simulink model "PubIfDecisionTOS_MDL"  (R2020b)
settings: configuration reference "DspaceConfig" (kept outside this file)
PostLoadFcn:
  | if any(exist('dsrtsu_mdlpostloadfcn', 'file') ~= 0), dsrtsu_mdlpostloadfcn('Execute', bdroot); end
InitFcn:
  | , if any(exist('dsmpb_private', 'file') ~= 0), dsmpb_private('dsmpb_mdlclblib', 'Init', bdroot); end,
undefined symbols (not defined in the file or in its folder): C_TOS_ACCEgoRAxletoFbumplength_m, C_TOS_ACCTargetFront_Flag, C_TOS_AEBJAPedObjDxThre_Val, C_TOS_AEBJAPedObjDyThre_Val, C_TOS_AEBJATargetSize_Val, C_TOS_AEBJAVehObjDxThre_Val, C_TOS_AEBJAVehObjDyThre_Val, C_TOS_AEBJuncPedTargetSize_Val, C_TOS_AEBLatObjDxThre_Val, C_TOS_AEBLatPedDyThre_Val, C_TOS_AEBLatTargetSize_Val, C_TOS_AEBLongTargetInEgoFront_Flag, C_TOS_axAbsGround_Parameter, C_TOS_CameraConfirmedFlag, C_TOS_CNsubjWidth, C_TOS_CurrentLaneCoreMinWidth_Val, C_TOS_CutInProb_Val_Zero, C_TOS_CutOutProb_Val_Zero, C_TOS_D2R_Val, C_TOS_DefaultValueObjectToCenterLine_dy, C_TOS_EgoCarWidth_Val, C_TOS_EgoDxRefPoint_m, C_TOS_EgoRAxletoFbumplength_m, C_TOS_HalfWidthVehicle_Con, C_TOS_HWA_CurrentLaneFlag, C_TOS_HWA_LeftLaneFlag, C_TOS_HWA_MovingDir_Vaild, C_TOS_HWA_MovState_Vaild, C_TOS_HWA_RightLaneFlag, C_TOS_LaneLineCourseErrorFront, C_TOS_LaneLineCourseErrorRear, C_TOS_MotorbikeDefaultWidth_m, C_TOS_NumberOfEffectiveTargets, C_TOS_Obj_Age_Val, C_TOS_Objdx_Constraint_Val, C_TOS_ObjectDefaultWidth_m, C_TOS_ObjInCurrentLane_Val, C_TOS_ObjInCurrentLaneValid, C_TOS_ObjInLeftLaneValid, C_TOS_ObjInRightLaneValid, C_TOS_ObjNotInCurrentLane_Val, C_TOS_ObjNotREElementType, C_TOS_ObjPredictDis_dy_ConstantVal_Zeros, C_TOS_ObjToCenterLine_ConstantVal_Zeros, C_TOS_OFMObjIDInvilad_Val, C_TOS_PIL_LatDisCons_Val_zero, C_TOS_PIL_ObjectCutInFlag_b, C_TOS_PIL_ObjectCutOutFlag_b, C_TOS_PIL_ObjLaneProb_al_Val, C_TOS_PP_ObjFusType_FC_Confirm_b, C_TOS_PP_ObjFusType_FC_FR_Confirm_b, C_TOS_PP_ObjFusType_FR_Confirm_b, C_TOS_RE_80BoolDefault_Val, C_TOS_RE_80Single181Default_Val, C_TOS_RE_80Single255Default_Val, C_TOS_RE_80Uint8Default_Val, C_TOS_RE_D2R, C_TOS_RE_D_180_Val, C_TOS_RE_InvalidObjectID_Val, C_TOS_RE_InvalidTargetChainDir_Val ... (+142)
libraries: simulink x1650, TOS_LIB x361, canfdmsglib x14
(part 6 of 69)

== system PubIfDecisionTOS_MDL/TOS_20201112/TOS_2012080320/PIL_1029/BoundaryCalculat/ObjectToCenterLine_dyc ==
  OFM_SignalVerification : Inport
  Left_CenterLine : Inport  Port=2
  Same_CenterLine : Inport  Port=3
  Right_CenterLine : Inport  Port=4
  Bus Creator1 : BusCreator  Inputs=4
  Bus Selector1 : BusSelector  OutputSignals=Left_CenterLine,OFM_SignalVerification
  Bus Selector2 : BusSelector  OutputSignals=Same_CenterLine,OFM_SignalVerification
  Bus Selector5 : BusSelector  OutputSignals=Right_CenterLine,OFM_SignalVerification
  LeftLane : Subsystem
  RightLane : Subsystem
  SameLane : Subsystem
  Terminator : Terminator
  Terminator1 : Terminator
  Terminator2 : Terminator
  PIL_LeftCenterLine_dyc_Filt : Outport
  PIL_SameCenterLine_dyc_Filt : Outport  Port=2
  PIL_RightCenterLine_dyc_Filt : Outport  Port=3
  wires:
  Left_CenterLine/1 -> Bus Creator1/2  "Left_CenterLine"
  Same_CenterLine/1 -> Bus Creator1/3  "Same_CenterLine"
  Bus Creator1/1 -> Bus Selector1/1, Bus Selector2/1, Bus Selector5/1
  Bus Selector2/1 -> SameLane/1(Same_CenterLine)  "<Same_CenterLine>"
  Bus Selector2/2 -> SameLane/2(OFM_SignalVerification)  "<OFM_SignalVerification>"
  SameLane/1(PIL_SameCenterLine_dyc) -> Terminator1/1  "PIL_SameCenterLine_dyc"
  LeftLane/1(PIL_LeftCenterLine_dyc) -> Terminator/1  "PIL_LeftCenterLine_dyc"
  Bus Selector1/1 -> LeftLane/1(Left_CenterLine)  "<Left_CenterLine>"
  Bus Selector1/2 -> LeftLane/2(OFM_SignalVerification)  "<OFM_SignalVerification>"
  RightLane/1(PIL_RightCenterLine_dyc) -> Terminator2/1  "PIL_RightCenterLine_dyc"
  Right_CenterLine/1 -> Bus Creator1/4  "Right_CenterLine"
  OFM_SignalVerification/1 -> Bus Creator1/1  "OFM_SignalVerification"
  Bus Selector5/2 -> RightLane/2(OFM_SignalVerification)  "<OFM_SignalVerification>"
  Bus Selector5/1 -> RightLane/1(CenterOfRightLane)  "<Right_CenterLine>"
  LeftLane/2(PIL_LeftCenterLine_dyc_Filt) -> PIL_LeftCenterLine_dyc_Filt/1
  SameLane/2(PIL_SameCenterLine_dyc_Filt) -> PIL_SameCenterLine_dyc_Filt/1
  RightLane/2(PIL_RightCenterLine_dyc_Filt) -> PIL_RightCenterLine_dyc_Filt/1

== system PubIfDecisionTOS_MDL/TOS_20201112/TOS_2012080320/PIL_1029/ObjCutInOut_Prob/ObjectCutIn ==
  TOS_OFMObjValid_Flag : Inport
  Object_Width : Inport  Port=2  OutDataTypeStr=single
  Object_DX : Inport  Port=3  OutDataTypeStr=single
  Object_DY : Inport  Port=4  OutDataTypeStr=single
  Object_Age : Inport  Port=5  OutDataTypeStr=uint16
  Object_Type : Inport  Port=6
  Object_MovingState : Inport  Port=7
  PP_ObjectToCenterLine_dy : Inport  Port=8  OutDataTypeStr=single
  PP_ObjectToCenterLine_vyc : Inport  Port=9  OutDataTypeStr=single
  PP_CurrentLaneWidth : Inport  Port=10
  PIL_ObjectToCenterLine_dy_Filt : Inport  Port=11  OutDataTypeStr=single
  Bus Creator : BusCreator  Inputs=11
  Bus Creator1 : BusCreator  Inputs=5
  Bus Selector : BusSelector  OutputSignals=TOS_OFMObjValid_Flag,Object_Width,Object_DX,Object_DY,Object_Age,Object_Type,PP_ObjectToCenterLine_dy,PP_ObjectToCenterLine_vyc,PIL_ObjectToCenterLine_dy_Filt,PP_CurrentLaneWidth
  Bus Selector4 : BusSelector  OutputSignals=Object_DX,TOS_OFMObjValid_Flag,Object_MovingState
  CutInProb_Calculate : Subsystem
  CutInProb_Pluse : Subsystem
  Terminator : Terminator
  Unit Delay : UnitDelay  InitialCondition=zeros(80,1)  SampleTime=-1  HasFrameUpgradeWarning=on
  TOS_PIL_ObjectCutInPro_Filt : Outport
  TOS_PIL_ObjectCutIn_Flag : Outport  Port=2
  wires:
  Bus Creator1/1 -> Terminator/1  "TOS_PIL_Cutin_ObserVale"
  Bus Selector4/3 -> CutInProb_Pluse/5(Object_MovingState)  "<Object_MovingState>"
  Object_MovingState/1 -> Bus Creator/7  "Object_MovingState"
  CutInProb_Pluse/1(PIL_CutInProb_Pluse) -> TOS_PIL_ObjectCutInPro_Filt/1, Unit Delay/1  "TOS_PIL_ObjectCutInPro_Filt"
  CutInProb_Pluse/2(PIL_ObjectCutInFlag) -> TOS_PIL_ObjectCutIn_Flag/1  "TOS_PIL_ObjectCutIn_Flag"
  Object_Width/1 -> Bus Creator/2  "Object_Width"
  Object_DX/1 -> Bus Creator/3  "Object_DX"
  Object_DY/1 -> Bus Creator/4  "Object_DY"
  Object_Age/1 -> Bus Creator/5  "Object_Age"
  PP_ObjectToCenterLine_dy/1 -> Bus Creator/8  "PP_ObjectToCenterLine_dy"
  PP_ObjectToCenterLine_vyc/1 -> Bus Creator/9  "PP_ObjectToCenterLine_vyc"
  PIL_ObjectToCenterLine_dy_Filt/1 -> Bus Creator/11  "PIL_ObjectToCenterLine_dy_Filt"
  Bus Creator/1 -> Bus Selector/1, [ObjCutInSig]
  Unit Delay/1 -> CutInProb_Pluse/1(CutInProb_Pluse_K1)
  Object_Type/1 -> Bus Creator/6  "Object_Type"
  PP_CurrentLaneWidth/1 -> Bus Creator/10  "PP_CurrentLaneWidth"
  Bus Selector4/1 -> CutInProb_Pluse/3(Object_Dx)  "<Object_DX>"
  [ObjCutInSig] -> Bus Selector4/1
  CutInProb_Calculate/5(CutInProb_Calculate) -> Bus Creator1/5, CutInProb_Pluse/2(CutInProb_ScopeConstraint)  "TOS_PIL_CutInProb_Calculate"
  Bus Selector/2 -> CutInProb_Calculate/2(Object_Width)  "<Object_Width>"
  Bus Selector/3 -> CutInProb_Calculate/3(Object_DX)  "<Object_DX>"
  Bus Selector/4 -> CutInProb_Calculate/4(Object_DY)  "<Object_DY>"
  Bus Selector/5 -> CutInProb_Calculate/5(Object_Age)  "<Object_Age>"
  Bus Selector/6 -> CutInProb_Calculate/6(Object_Type)  "<Object_Type>"
  Bus Selector/7 -> CutInProb_Calculate/7(PP_ObjectToCenterLine_dy)  "<PP_ObjectToCenterLine_dy>"
  Bus Selector/8 -> CutInProb_Calculate/8(PP_ObjectToCenterLine_vyc)  "<PP_ObjectToCenterLine_vyc>"
  Bus Selector/9 -> CutInProb_Calculate/9(PIL_ObjectToCenterLine_dy_Filt)  "<PIL_ObjectToCenterLine_dy_Filt>"
  Bus Selector/10 -> CutInProb_Calculate/10(PP_CurrentLaneWidth)  "<PP_CurrentLaneWidth>"
  CutInProb_Calculate/1(PIL_CutInPredictTime_ObserVale) -> Bus Creator1/1  "TOS_PIL_CutInPredictTime_ObserVale"
  CutInProb_Calculate/2(PIL_CutInPredictTime_dxConstraint_ObserVale) -> Bus Creator1/2  "TOS_PIL_CutInPredictTime_dxConstraint_ObserVale"
  CutInProb_Calculate/3(PIL_CutInPredictDis_dy_ObjWidthConstraint_ObserVale) -> Bus Creator1/3  "TOS_PIL_CutInPredictDis_dy_ObjWidthConstraint_ObserVale"
  CutInProb_Calculate/4(PIL_ObjectCutinMindFlg_ObserVale) -> Bus Creator1/4  "TOS_PIL_CutinMindFlg_ObserVale"
  TOS_OFMObjValid_Flag/1 -> Bus Creator/1  "TOS_OFMObjValid_Flag"
  Bus Selector/1 -> CutInProb_Calculate/1(TOS_OFMObjValid_Flag)  "<TOS_OFMObjValid_Flag>"
  Bus Selector4/2 -> CutInProb_Pluse/4(TOS_OFMObjValid_Flag)  "<TOS_OFMObjValid_Flag>"

== system PubIfDecisionTOS_MDL/TOS_20201112/TOS_2012080320/PIL_1029/ObjCutInOut_Prob/ObjectCutOut ==
  TOS_OFMObjValid_Flag : Inport
  Object_Width : Inport  Port=2
  Object_DX : Inport  Port=3
  Object_DY : Inport  Port=4
  Object_Age : Inport  Port=5
  Object_Type : Inport  Port=6
  Object_MovingState : Inport  Port=7
  Object_VY : Inport  Port=8
  Object_Std_DY : Inport  Port=9
  PP_ObjectToCenterLine_dy : Inport  Port=10
  PP_ObjectToCenterLine_vyc : Inport  Port=11
  PIL_ObjectToCenterLine_dy_Filt : Inport  Port=12
  Bus Creator : BusCreator  Inputs=11
  Bus Creator1 : BusCreator  Inputs=7
  Bus Selector : BusSelector  OutputSignals=TOS_OFMObjValid_Flag,Object_Width,Object_DX,Object_DY,Object_Age,Object_Type,PP_ObjectToCenterLine_dy,PP_ObjectToCenterLine_vyc,PIL_ObjectToCenterLine_dy_Filt,Object_VY
  Bus Selector4 : BusSelector  OutputSignals=TOS_OFMObjValid_Flag,Object_MovingState
  CutOutProb_Calculate : Subsystem
  CutOutProb_Pluse : Subsystem
  Subsystem : Subsystem
  Terminator : Terminator
  Terminator1 : Terminator
  Unit Delay : UnitDelay  InitialCondition=zeros(80,1)  SampleTime=-1  HasFrameUpgradeWarning=on
      settings: AttributesFormatString=initVal = zeros(80,1)
  TOS_PIL_ObjectCutOutPro_Filt : Outport
  TOS_PIL_ObjectCutOut_Flag : Outport  Port=2
  wires:
  Subsystem/1(Out1) -> CutOutProb_Calculate/10(Object_VY)  "OBJ_VY"
  Bus Selector/10 -> Subsystem/1(In1)  "<Object_VY>"
  Object_VY/1 -> Bus Creator/11  "Object_VY"
  Bus Selector4/2 -> CutOutProb_Pluse/4(Object_MovingState)  "<Object_MovingState>"
  Object_MovingState/1 -> Bus Creator/10  "Object_MovingState"
  Unit Delay/1 -> CutOutProb_Pluse/1(CutOutProb_Pluse_K1)
  CutOutProb_Pluse/2(PIL_ObjectCutOutFlag) -> TOS_PIL_ObjectCutOut_Flag/1  "TOS_PIL_ObjectCutOut_Flag"
  CutOutProb_Pluse/1(PIL_CutOutProb_Pluse) -> Unit Delay/1, TOS_PIL_ObjectCutOutPro_Filt/1  "TOS_PIL_ObjectCutOutPro_Filt"
  CutOutProb_Calculate/1(PIL_CutOutPredictTime_ObserVale) -> Bus Creator1/1  "TOS_PIL_CutOutPredictTime_ObserVale"
  CutOutProb_Calculate/2(PIL_CutOutPredictTime_dxConstraint_ObserVale) -> Bus Creator1/2  "TOS_PIL_CutOutPredictTime_dxConstraint_ObserVale"
  CutOutProb_Calculate/3(PIL_CutOutPredictDis_dy_ObjWidthConstraint_ObserVale) -> Bus Creator1/3  "TOS_CutOutPredictDis_dy_ObjWidthConstraint_ObserVale"
  CutOutProb_Calculate/4(PIL_ObjectCutOutMindFlg_ObserVale) -> Bus Creator1/4  "TOS_PIL_ObjectCutOutMindFlg_ObserVale"
  CutOutProb_Calculate/8(PIL_CutOutProb_ScopeConstraint) -> CutOutProb_Pluse/2(CutOutProb_ScopeConstraint)
  Bus Creator/1 -> Bus Selector/1, [ObjectCutOut]
  TOS_OFMObjValid_Flag/1 -> Bus Creator/1  "TOS_OFMObjValid_Flag"
  Object_Width/1 -> Bus Creator/2  "Object_Width"
  Object_DX/1 -> Bus Creator/3  "Object_DX"
  Object_DY/1 -> Bus Creator/4  "Object_DY"
  Object_Age/1 -> Bus Creator/5  "Object_Age"
  Object_Type/1 -> Bus Creator/6  "Object_Type"
  PP_ObjectToCenterLine_dy/1 -> Bus Creator/7  "PP_ObjectToCenterLine_dy"
  PP_ObjectToCenterLine_vyc/1 -> Bus Creator/8  "PP_ObjectToCenterLine_vyc"
  PIL_ObjectToCenterLine_dy_Filt/1 -> Bus Creator/9  "PIL_ObjectToCenterLine_dy_Filt"
  Bus Selector/1 -> CutOutProb_Calculate/1(TOS_OFMObjValid_Flag)  "<TOS_OFMObjValid_Flag>"
  Bus Selector/2 -> CutOutProb_Calculate/2(Object_Width)  "<Object_Width>"
  Bus Selector/3 -> CutOutProb_Calculate/3(Object_DX)  "<Object_DX>"
  Bus Selector/4 -> CutOutProb_Calculate/4(Object_DY)  "<Object_DY>"
  Bus Selector/5 -> CutOutProb_Calculate/5(Object_Age)  "<Object_Age>"
  Bus Selector/6 -> CutOutProb_Calculate/6(Object_Type)  "<Object_Type>"
  Bus Selector/7 -> CutOutProb_Calculate/7(PP_ObjectToCenterLine_dy)  "<PP_ObjectToCenterLine_dy>"
  Bus Selector/8 -> CutOutProb_Calculate/8(PP_ObjectToCenterLine_vyc)  "<PP_ObjectToCenterLine_vyc>"
  Bus Selector/9 -> CutOutProb_Calculate/9(PIL_ObjectToCenterLine_dy_Filt)  "<PIL_ObjectToCenterLine_dy_Filt>"
  [ObjectCutOut] -> Bus Selector4/1
  Bus Selector4/1 -> CutOutProb_Pluse/3(TOS_OFMObjValid_Flag)  "<TOS_OFMObjValid_Flag>"
  Object_Std_DY/1 -> Terminator/1
  CutOutProb_Calculate/5(PIL_ObjectCutoutMindFlg1_ObserVale) -> Bus Creator1/5  "TOS_PIL_ObjectCutoutMindFlg1_ObserVale"
  CutOutProb_Calculate/6(PIL_ObjectCutoutMindFlg2_ObserVale) -> Bus Creator1/6  "TOS_PIL_ObjectCutoutMindFlg2_ObserVale"
  CutOutProb_Calculate/7(PIL_ObjectCutoutMindFlg3_ObserVale) -> Bus Creator1/7  "TOS_PIL_ObjectCutoutMindFlg3_ObserVale"
  Bus Creator1/1 -> Terminator1/1  "TOS_PIL_CutOut_ObserVale"

== system PubIfDecisionTOS_MDL/TOS_20201112/TOS_2012080320/PIL_1029/OverlapRatio_Calculate/OverlapCalculation_Default ==
  Action Port : ActionPort  ActionPortLabel=if(u1 ~= 0)
  Constant2 : Constant  Value=0  OutDataTypeStr=single
  PIL_overlapRatio : Outport  OutDataTypeStr=single
  wires:
  Constant2/1 -> PIL_overlapRatio/1

== system PubIfDecisionTOS_MDL/TOS_20201112/TOS_2012080320/PIL_1029/OverlapRatio_Calculate/PIL_OverlapCalculation ==
  ObjectWidth : Inport
  ObjectTypeCameraConfirmed : Inport  Port=2
  object_MovingState : Inport  Port=3
  Object_Type : Inport  Port=4
  dyEgo2Center : Inport  Port=5
  dyObject2Center : Inport  Port=6
  Action Port : ActionPort  ActionPortLabel=else
  OverlapRatioCalcFlow : Stateflow chart  TreatAsAtomicUnit=on
  TargetWidthCalc : Subsystem
  dyCriticalEgoObjCalc : Subsystem
  overlapRatio : Outport
  wires:
  dyObject2Center/1 -> OverlapRatioCalcFlow/3(dyObject2Center)
  dyEgo2Center/1 -> OverlapRatioCalcFlow/2(dyEgo2Center)
  OverlapRatioCalcFlow/1(overlapRatio) -> overlapRatio/1
  dyCriticalEgoObjCalc/1(dyCriticalEgoObj) -> OverlapRatioCalcFlow/1(dyCriticalEgoObj)  "dyCriticalEgoObj"
  TargetWidthCalc/1(objWidth) -> dyCriticalEgoObjCalc/1(objWidth)  "objWidth"
  object_MovingState/1 -> TargetWidthCalc/3(object_MovingState)
  ObjectTypeCameraConfirmed/1 -> TargetWidthCalc/2(ObjectTypeCameraConfirmed)
  ObjectWidth/1 -> TargetWidthCalc/1(ObjectWidth)
  Object_Type/1 -> TargetWidthCalc/4(Object_Type)

== system PubIfDecisionTOS_MDL/TOS_20201112/TOS_2012080320/PIL_1029/PIL_ObjectToCenterLine_dy_Filt/PIL_ObjectToCenterLine_dy ==
  ObjectID_Filt_K1 : Inport
  ObjectToCenterLine_dy_Filt_K1 : Inport  Port=2  OutDataTypeStr=single
  ObjectToCenterLine_dy : Inport  Port=3  OutDataTypeStr=single  Partition=on  PartitionDimension=1  PartitionWidth=1  PartitionOffset=0
  TOS_OFMObjValid_Flag : Inport  Port=4  OutDataTypeStr=uint8  Partition=on  PartitionDimension=1  PartitionWidth=1  PartitionOffset=0
  Object_ID : Inport  Port=5  OutDataTypeStr=uint8  Partition=on  PartitionDimension=1  PartitionWidth=1  PartitionOffset=0
  Object_Age : Inport  Port=6  Partition=on  PartitionDimension=1  PartitionWidth=1  PartitionOffset=0
  Compare To Constant : simulink/Logic and Bit Operations/Compare To Constant  relop===  const=C_TOS_OFMObjIDInvilad_Val  OutDataTypeStr=boolean
      settings: AttributesFormatString=C_TOS_OFMObjIDInvilad_Val = 0
  For Each : ForEach  DisableCoverage=on
  If : If  IfExpression=u1 ~= 0
  Merge : Merge
  Merge1 : Merge
  PP_SignalProcessingDefault : Subsystem  TreatAsAtomicUnit=on
  Subsystem : Subsystem
  Obj_ID : Outport  ConcatenationDimension=1
  ObjectToCenterLine_dy_Filt : Outport  Port=2  OutDataTypeStr=single  ConcatenationDimension=1
  wires:
  [TOS_OFMObjValid_Flag] -> Subsystem/6(TOS_OFMObjValid_Flag)
  TOS_OFMObjValid_Flag/1 -> Compare To Constant/1, [TOS_OFMObjValid_Flag]
  Object_Age/1 -> Subsystem/5(Object_Age)
  Merge/1 -> Obj_ID/1
  Merge1/1 -> ObjectToCenterLine_dy_Filt/1
  PP_SignalProcessingDefault/2(ObjectToCenterLine_dy_Filt) -> Merge1/1
  PP_SignalProcessingDefault/1(Obj_ID) -> Merge/1
  Subsystem/2(ObjectToCenterLine_dy_Filt) -> Merge1/2
  Subsystem/1(Obj_ID) -> Merge/2
  ObjectToCenterLine_dy/1 -> Subsystem/3(ObjectToCenterLine_dy)
  ObjectToCenterLine_dy_Filt_K1/1 -> Subsystem/2(ObjectToCenterLine_dy_Filt_K1)
  ObjectID_Filt_K1/1 -> Subsystem/1(ObjectID_Filt_K1)
  Compare To Constant/1 -> If/1
  Object_ID/1 -> Subsystem/4(Object_ID)
  If/1 -> PP_SignalProcessingDefault/Action
  If/2 -> Subsystem/Action

== system PubIfDecisionTOS_MDL/TOS_20201112/TOS_2012080320/PIL_1029/ProbCalculat/ProbCalculat ==
  OFM_SignalVerification : Inport
  CurrentLane_Boundary : Inport  Port=2
  PIL_ObjectToCenterLine_dyc : Inport  Port=3
  LM_SignalVerification : Inport  Port=4
  Bus Selector1 : BusSelector  OutputSignals=PIL_SameCenterLine_dyc,PIL_LeftCenterLine_dyc,PIL_RightCenterLine_dyc
  Bus Selector2 : BusSelector  OutputSignals=SameLane_CoreArea_Boundary,SameLane_EdgeLeft_Boundary,SameLane_EdgeRight_Boundary,LeftLane_CoreArea_Boundary,LeftLane_EdgeLeft_Boundary,LeftLane_EdgeRight_Boundary,RightLane_CoreArea_Boundary,RightLane_EdgeLeft_Boundary,RightLane_EdgeRight_Boundary
  Bus Selector3 : BusSelector  OutputSignals=TOS_OFMObjValid_Flag,Object_Width,Object_Type
  ObjectProbCalculation : Subsystem
  Subsystem : Subsystem
  PIL_EgoLaneProb : Outport  InitialOutput=0
  PIL_LeftLaneProb : Outport  Port=2
  PIL_RightLaneProb : Outport  Port=3
  "PIL_ObjLaneProb_all " : Outport  Port=4  InitialOutput=0
  PIL_EgoVehicleProFilt : Outport  Port=5
  wires:
  Bus Selector2/9 -> ObjectProbCalculation/15(RightLane_EdgeRight_Boundary)  "<RightLane_EdgeRight_Boundary>"
  Bus Selector2/8 -> ObjectProbCalculation/14(RightLane_EdgeLeft_Boundary)  "<RightLane_EdgeLeft_Boundary>"
  Bus Selector2/7 -> ObjectProbCalculation/13(RightLane_CoreArea_Boundary)  "<RightLane_CoreArea_Boundary>"
  Bus Selector2/6 -> ObjectProbCalculation/12(LeftLane_EdgeRight_Boundary)  "<LeftLane_EdgeRight_Boundary>"
  Bus Selector2/5 -> ObjectProbCalculation/11(LeftLane_EdgeLeft_Boundary)  "<LeftLane_EdgeLeft_Boundary>"
  Bus Selector2/4 -> ObjectProbCalculation/10(LeftLane_CoreArea_Boundary)  "<LeftLane_CoreArea_Boundary>"
  Bus Selector1/3 -> ObjectProbCalculation/6(PIL_RightCenterLine_dyc)  "<PIL_RightCenterLine_dyc>"
  Bus Selector1/2 -> ObjectProbCalculation/5(PIL_LeftCenterLine_dyc)  "<PIL_LeftCenterLine_dyc>"
  Bus Selector1/1 -> ObjectProbCalculation/4(PIL_SameCenterLine_dyc)  "<PIL_SameCenterLine_dyc>"
  PIL_ObjectToCenterLine_dyc/1 -> Bus Selector1/1
  Bus Selector2/2 -> ObjectProbCalculation/8(SameLane_EdgeLeft_Boundary)  "<SameLane_EdgeLeft_Boundary>"
  Bus Selector2/3 -> ObjectProbCalculation/9(SameLane_EdgeRight_Boundary)  "<SameLane_EdgeRight_Boundary>"
  Bus Selector2/1 -> ObjectProbCalculation/7(SameLane_CoreArea_Boundary)  "<SameLane_CoreArea_Boundary>"
  Bus Selector3/3 -> ObjectProbCalculation/3(Object_Type)  "<Object_Type>"
  Bus Selector3/2 -> ObjectProbCalculation/2(Object_Width)  "<Object_Width>"
  Bus Selector3/1 -> ObjectProbCalculation/1(TOS_OFMObjValid_Flag)  "<TOS_OFMObjValid_Flag>"
  CurrentLane_Boundary/1 -> Bus Selector2/1
  OFM_SignalVerification/1 -> Bus Selector3/1
  LM_SignalVerification/1 -> Subsystem/1(LM_SignalVerification)
  Subsystem/1(PIL_EgoVehicleProFilt) -> PIL_EgoVehicleProFilt/1
  ObjectProbCalculation/1("PIL_ObjLaneProb_all ") -> "PIL_ObjLaneProb_all "/1  "PIL_ObjLaneProb_all"
  ObjectProbCalculation/2(PIL_EgoLaneProb) -> PIL_EgoLaneProb/1  "PIL_EgoLaneProb"
  ObjectProbCalculation/3(PIL_LeftLaneProb) -> PIL_LeftLaneProb/1  "PIL_LeftLaneProb"
  ObjectProbCalculation/4(PIL_RightLaneProb) -> PIL_RightLaneProb/1  "PIL_RightLaneProb"

== system PubIfDecisionTOS_MDL/TOS_20201112/TOS_2012080320/PIL_1029/ProbCalculat/ProbFilt ==
  OFM_InPutSig : Inport
  PIL_ObjinEgoLaneProb : Inport  Port=2
  PIL_ObjinLeftLaneProb : Inport  Port=3
  PIL_ObjinRightLaneProb : Inport  Port=4
  ObjinEgoLaneProb : Subsystem
  ObjinLeftLaneProb : Subsystem
  ObjinRightLaneProb : Subsystem
  Signal Copy : SignalConversion  OverrideOpt=off
  Signal Copy1 : SignalConversion  OverrideOpt=off
  Signal Copy2 : SignalConversion  OverrideOpt=off
  Terminator : Terminator
  PIL_ObjinEgoLaneProb_Filt : Outport
  PIL_ObjinLeftLaneProb_Filt : Outport  Port=2
  PIL_ObjinRightLaneProb_Filt : Outport  Port=3
  wires:
  ObjinRightLaneProb/1(PIL_ObjinRightLaneProb_Filt) -> Signal Copy/1
  ObjinLeftLaneProb/1(PIL_ObjinLeftLaneProb_Filt) -> Signal Copy1/1
  ObjinEgoLaneProb/1(PIL_ObjinEgoLaneProb_Filt) -> Signal Copy2/1
  Signal Copy/1 -> PIL_ObjinRightLaneProb_Filt/1  "TOS_PIL_RightLaneProb_Filt"
  Signal Copy1/1 -> PIL_ObjinLeftLaneProb_Filt/1  "TOS_PIL_LeftLaneProb_Filt"
  Signal Copy2/1 -> PIL_ObjinEgoLaneProb_Filt/1  "TOS_PIL_SameLanePro_Filt"
  PIL_ObjinEgoLaneProb/1 -> ObjinEgoLaneProb/1(PIL_ObjinEgoLaneProb)
  PIL_ObjinLeftLaneProb/1 -> ObjinLeftLaneProb/1(PIL_ObjinLeftLaneProb)
  PIL_ObjinRightLaneProb/1 -> ObjinRightLaneProb/1(PIL_ObjinRightLaneProb)
  OFM_InPutSig/1 -> Terminator/1

== system PubIfDecisionTOS_MDL/TOS_20201112/TOS_2012080320/PP1128/AAT-AdditionalAttributes/PP_CenterLine_Calculat ==
  OFM_SignalVerification : Inport
  LM_SignalVerification : Inport  Port=2
  EgoLane_CenterLine : Subsystem
  LaneWidth : Subsystem
  LaneWidth_80 : Subsystem  Commented=on
  LeftLane_CenterLine : Subsystem
  RightLane_CenterLine : Subsystem
  Terminator : Terminator  Commented=on
  PP_EgoLane_CenterLine : Outport
  PP_LeftLane_CenterLine : Outport  Port=2
  PP_RightLane_CenterLine : Outport  Port=3
  PP_LaneWidth : Outport  Port=4
  wires:
  LM_SignalVerification/1 -> EgoLane_CenterLine/1(EgoLane), RightLane_CenterLine/1(LeftLane), LeftLane_CenterLine/1(LeftLane), LaneWidth/1(LM_SignalVerification), LaneWidth_80/2(LM_SignalVerification)
  EgoLane_CenterLine/1(PP_EgoLane_CenterLine) -> PP_EgoLane_CenterLine/1
  LeftLane_CenterLine/1(PP_LeftLane_CenterLine) -> PP_LeftLane_CenterLine/1
  RightLane_CenterLine/1(PP_RightLane_CenterLine) -> PP_RightLane_CenterLine/1
  LaneWidth/1(PP_LaneWidth) -> PP_LaneWidth/1
  OFM_SignalVerification/1 -> LaneWidth_80/1(OFM_SignalVerification)
  LaneWidth_80/1(PP_LaneWidth) -> Terminator/1

== system PubIfDecisionTOS_MDL/TOS_20201112/TOS_2012080320/PP1128/AAT-AdditionalAttributes/PP_ObjFirstDxDyDetermineSignalProcessing ==
  Object_DX : Inport
  Object_DY : Inport  Port=2
  Object_ID : Inport  Port=3
  TOS_OFMObjValid_Flag : Inport  Port=4
  PP_ObjFirstDxDyDetermine : Subsystem
  Unit Delay : UnitDelay  InitialCondition=zeros(80,1)  SampleTime=-1  HasFrameUpgradeWarning=on
      settings: AttributesFormatString=initVal = zeros(80,1)
  Unit Delay1 : UnitDelay  InitialCondition=zeros(80,1)  SampleTime=-1  HasFrameUpgradeWarning=on
      settings: AttributesFormatString=initVal = zeros(80,1)
  Unit Delay2 : UnitDelay  InitialCondition=zeros(80,1)  SampleTime=-1  HasFrameUpgradeWarning=on
      settings: AttributesFormatString=initVal = zeros(80,1)
  PP_ObjFirstDetect_Dx : Outport
  PP_ObjFirstDetect_Dy : Outport  Port=2
  wires:
  Unit Delay2/1 -> PP_ObjFirstDxDyDetermine/1(Object_ID_Last)
  PP_ObjFirstDxDyDetermine/3(PP_ObjFirstDetect_Dy) -> Unit Delay/1, PP_ObjFirstDetect_Dy/1
  PP_ObjFirstDxDyDetermine/1(Object_ID_temp) -> Unit Delay2/1
  Unit Delay/1 -> PP_ObjFirstDxDyDetermine/3(Object_Dy_Last)
  PP_ObjFirstDxDyDetermine/2(PP_ObjFirstDetect_Dx) -> Unit Delay1/1, PP_ObjFirstDetect_Dx/1
  Unit Delay1/1 -> PP_ObjFirstDxDyDetermine/2(Object_Dx_Last)
  Object_DX/1 -> PP_ObjFirstDxDyDetermine/4(Object_Dx)
  Object_DY/1 -> PP_ObjFirstDxDyDetermine/5(Object_Dy)
  Object_ID/1 -> PP_ObjFirstDxDyDetermine/6(Object_ID)
  TOS_OFMObjValid_Flag/1 -> PP_ObjFirstDxDyDetermine/7(TOS_OFMObjValid_Flag)

== system PubIfDecisionTOS_MDL/TOS_20201112/TOS_2012080320/PP1128/AAT-AdditionalAttributes/PP_ObjectToCenterLine_dy ==
  "OFM_SignalVerification " : Inport
  LM_SignalVerification : Inport  Port=2
  vxvRefMs : Inport  Port=3
  Bus Creator2 : BusCreator  Inputs=3
  Bus Selector2 : BusSelector  OutputSignals=LM_SignalVerification
  Bus Selector3 : BusSelector  OutputSignals=vxvRefMs,OFM_SignalVerification
  EgoLaneCenterLine : Subsystem
  PP_EgoVeh_Object_ToCenterLine : Subsystem
  PP_ObjectToCenterLine_vyc : Subsystem
  PP_EgoVehCenterLine_dy : Outport
  PP_ObjectToCenterLine_dy : Outport  Port=2
  PP_ObjectToCenterLine_Vyc : Outport  Port=3
  wires:
  PP_EgoVeh_Object_ToCenterLine/2(PP_ObjectToCenterLine_dy) -> PP_ObjectToCenterLine_dy/1
  PP_EgoVeh_Object_ToCenterLine/1(PP_EgoVehCenterLine_dy) -> PP_EgoVehCenterLine_dy/1
  EgoLaneCenterLine/1(EgoLaneCenterLine) -> PP_ObjectToCenterLine_vyc/3(EgoLaneCenterLine), PP_EgoVeh_Object_ToCenterLine/2(EgoLaneCenterLine)
  Bus Creator2/1 -> Bus Selector2/1, [OFM_SignalVerification], Bus Selector3/1
  Bus Selector3/2 -> PP_EgoVeh_Object_ToCenterLine/1(OFM_SignalVerification), PP_ObjectToCenterLine_vyc/2(OFM_SignalVerification)  "<OFM_SignalVerification>"
  "OFM_SignalVerification "/1 -> Bus Creator2/1  "OFM_SignalVerification"
  LM_SignalVerification/1 -> Bus Creator2/2  "LM_SignalVerification"
  Bus Selector2/1 -> EgoLaneCenterLine/1(LM_SignalVerification)  "<LM_SignalVerification>"
  PP_ObjectToCenterLine_vyc/1(PP_ObjectToCenterLine_vyc) -> PP_ObjectToCenterLine_Vyc/1  "PP_ObjectToCenterLine_vyc"
  vxvRefMs/1 -> Bus Creator2/3  "vxvRefMs"
  Bus Selector3/1 -> PP_ObjectToCenterLine_vyc/1(vxvRefMs)  "<vxvRefMs>"

== system PubIfDecisionTOS_MDL/TOS_20201112/TOS_2012080320/PP1128/AAT-AdditionalAttributes/PP_SignalProcessing ==
  Object_MovingState : Inport  Partition=on  PartitionDimension=1  PartitionWidth=1  PartitionOffset=0
  Object_Orientation : Inport  Port=2  Partition=on  PartitionDimension=1  PartitionWidth=1  PartitionOffset=0
  Object_AX : Inport  Port=3  Partition=on  PartitionDimension=1  PartitionWidth=1  PartitionOffset=0
  axvRefMs2 : Inport  Port=4
  Object_MovingState1 : Inport  Port=5  Partition=on  PartitionDimension=1  PartitionWidth=1  PartitionOffset=0
  Object_Fus_Type : Inport  Port=6  Partition=on  PartitionDimension=1  PartitionWidth=1  PartitionOffset=0
  Object_DX : Inport  Port=7  Partition=on  PartitionDimension=1  PartitionWidth=1  PartitionOffset=0
  TOS_OFMObjValid_Flag : Inport  Port=8  Partition=on  PartitionDimension=1  PartitionWidth=1  PartitionOffset=0
  Compare To Constant : simulink/Logic and Bit Operations/Compare To Constant  relop===  const=C_TOS_OFMObjIDInvilad_Val  OutDataTypeStr=boolean
      settings: AttributesFormatString=C_TOS_OFMObjIDInvilad_Val = 0
  For Each : ForEach  DisableCoverage=on
  If : If  IfExpression=u1 ~= 0
  Merge{,1..8} (9 alike) : Merge
  PP_SignalProcessing : Subsystem  TreatAsAtomicUnit=on
  PP_SignalProcessingDefault : Subsystem  TreatAsAtomicUnit=on
  PP_MovingStateSignalProcessing : Outport  ConcatenationDimension=1
  PP_MovingState_AEB_SignalProcessing : Outport  Port=2  ConcatenationDimension=1
  PP_ObjMovingDirSignalProcessing : Outport  Port=3  ConcatenationDimension=1
  PP_axAbsGround : Outport  Port=4  ConcatenationDimension=1
  PP_CamareConfirmSignalProcessing : Outport  Port=5  ConcatenationDimension=1
  PP_ObjToEgoCarFrontbump : Outport  Port=6  ConcatenationDimension=1
  PP_ObjFusType_FC_FR_Confirm : Outport  Port=7  ConcatenationDimension=1
  PP_ObjFusType_FR_Confirm : Outport  Port=8  ConcatenationDimension=1
  PP_ObjFusType_FC_Confirm : Outport  Port=9  ConcatenationDimension=1
  wires:
  TOS_OFMObjValid_Flag/1 -> Compare To Constant/1
  Compare To Constant/1 -> If/1
  If/1 -> PP_SignalProcessingDefault/Action
  If/2 -> PP_SignalProcessing/Action
  Object_MovingState/1 -> PP_SignalProcessing/1(Object_MovingState)
  Object_Orientation/1 -> PP_SignalProcessing/2(Object_Orientation)
  Object_AX/1 -> PP_SignalProcessing/3(Object_AX)
  axvRefMs2/1 -> PP_SignalProcessing/4(axvRefMs2)
  Object_MovingState1/1 -> PP_SignalProcessing/5(Object_MovingState1)
  Object_Fus_Type/1 -> PP_SignalProcessing/6(Object_Fus_Type)
  Object_DX/1 -> PP_SignalProcessing/7(Object_DX)
  PP_SignalProcessing/1(PP_MovingStateSignalProcessing) -> Merge/2
  PP_SignalProcessing/3(PP_ObjMovingDirSignalProcessing) -> Merge1/2
  PP_SignalProcessing/4(PP_axAbsGround) -> Merge2/2
  PP_SignalProcessing/5(PP_CamareConfirmSignalProcessing) -> Merge3/2
  PP_SignalProcessing/6(PP_ObjToEgoCarFrontbump) -> Merge4/2
  Merge/1 -> PP_MovingStateSignalProcessing/1
  Merge1/1 -> PP_ObjMovingDirSignalProcessing/1
  Merge2/1 -> PP_axAbsGround/1
  Merge3/1 -> PP_CamareConfirmSignalProcessing/1
  Merge4/1 -> PP_ObjToEgoCarFrontbump/1
  PP_SignalProcessing/7(PP_ObjFusType_FC_FR_Confirm) -> Merge5/2
  PP_SignalProcessing/8(PP_ObjFusType_FR_Confirm) -> Merge6/2
  PP_SignalProcessing/9(PP_ObjFusType_FC_Confirm) -> Merge7/2
  Merge5/1 -> PP_ObjFusType_FC_FR_Confirm/1
  Merge7/1 -> PP_ObjFusType_FC_Confirm/1
  Merge6/1 -> PP_ObjFusType_FR_Confirm/1
  PP_SignalProcessing/2(PP_MovingState_AEB_SignalProcessing) -> Merge8/2
  Merge8/1 -> PP_MovingState_AEB_SignalProcessing/1
  PP_SignalProcessingDefault/1(PP_MovingStateSignalProcessing) -> Merge/1
  PP_SignalProcessingDefault/2(PP_MovingState_AEB_SignalProcessing) -> Merge8/1
  PP_SignalProcessingDefault/3(PP_ObjMovingDirSignalProcessing) -> Merge1/1
  PP_SignalProcessingDefault/4(PP_axAbsGround) -> Merge2/1
  PP_SignalProcessingDefault/5(PP_CamareConfirmSignalProcessing) -> Merge3/1
  PP_SignalProcessingDefault/6(PP_ObjToEgoCarFrontbump) -> Merge4/1
  PP_SignalProcessingDefault/7(PP_ObjFusType_FC_FR_Confirm) -> Merge5/1
  PP_SignalProcessingDefault/8(PP_ObjFusType_FR_Confirm) -> Merge6/1
  PP_SignalProcessingDefault/9(PP_ObjFusType_FC_Confirm) -> Merge7/1

== system PubIfDecisionTOS_MDL/TOS_20201112/TOS_2012080320/PP1128/AAT-AdditionalAttributes/RoadEdge ==
  OFM_SignalVerification : Inport
  LM_SignalVerification : Inport  Port=2
  VIE_SignalVerification : Inport  Port=3
  Bus Selector : BusSelector  OutputSignals=vxvRefMs
  Goto19 : Goto  Commented=on  GotoTag=RE_EdgeElementType
  Goto21 : Goto  Commented=on  GotoTag=RE_EgoRightStationaryObjectsSortIndex
  Goto22 : Goto  Commented=on  GotoTag=RE_StationaryObjectFlag
  Goto23 : Goto  Commented=on  GotoTag=RE_EgoLeftTargetChainStartIndex
  Goto24 : Goto  Commented=on  GotoTag=RE_EgoRightTargetChainStartIndex
  Goto25 : Goto  Commented=on  GotoTag=RE_EgoLeftEdgeGroupChainStartIndex
  Goto26 : Goto  Commented=on  GotoTag=RE_EgoRightEdgeGroupChainStartIndex
  Goto27 : Goto  Commented=on  GotoTag=RE_EgoLeftStationaryObjectsSortIndex
  RE_2020_12_07 : Subsystem
  Terminator : Terminator
  Terminator14 : Terminator
  RE_EdgeElementType : Outport
  wires:
  RE_2020_12_07/9(RE_EdgeElementID) -> Terminator14/1
  RE_2020_12_07/7(RE_EgoLeftStationaryObjectsSortIndex) -> Goto27/1
  RE_2020_12_07/8(RE_EgoRightStationaryObjectsSortIndex) -> Goto21/1
  RE_2020_12_07/1(RE_EdgeElementType) -> RE_EdgeElementType/1, Goto19/1
  RE_2020_12_07/2(RE_StationaryObjectFlag) -> Goto22/1
  LM_SignalVerification/1 -> Terminator/1
  RE_2020_12_07/4(RE_EgoRightTargetChainStartIndex) -> Goto24/1
  Bus Selector/1 -> RE_2020_12_07/2(vxvRefMs)  "<vxvRefMs>"
  VIE_SignalVerification/1 -> Bus Selector/1  "VIE_BUS"
  RE_2020_12_07/5(RE_EgoLeftEdgeGroupChainStartIndex) -> Goto25/1
  OFM_SignalVerification/1 -> RE_2020_12_07/1(OFM_OBJS), [OFM_SignalVerification]
  RE_2020_12_07/3(RE_EgoLeftTargetChainStartIndex) -> Goto23/1
  RE_2020_12_07/6(RE_EgoRightEdgeGroupChainStartIndex) -> Goto26/1

== system PubIfDecisionTOS_MDL/TOS_20201112/TOS_2012080320/PP1128/AAT-AdditionalAttributes/TAP_TargetPreprocessing ==
  OFM_Info : Inport
  OFM_SignalMaping : Subsystem
  TargetValidConfirm : Subsystem
  OFM_SignalVerification : Outport
  wires:
  TargetValidConfirm/1(TOS_OFMObjValid_Flag) -> OFM_SignalMaping/1(TOS_OFMObjValid_Flag)  "TOS_PP_TPA_OFMObjValid_Flag"
  OFM_SignalMaping/1(OFM_SignalVerification) -> OFM_SignalVerification/1
  OFM_Info/1 -> TargetValidConfirm/1(OFM_Info), OFM_SignalMaping/2(OFMInfo)

== system PubIfDecisionTOS_MDL/TOS_20201112/TOS_2012080320/PP1128/ISV_InputSignalVerification/LM_SignalVerif ==
  LM_LINE_LL : Inport  BusOutputAsStruct=on
  LM_LINE_LR : Inport  Port=2  BusOutputAsStruct=on
  LM_LINE_RL : Inport  Port=3  BusOutputAsStruct=on
  LM_LINE_RR : Inport  Port=4  BusOutputAsStruct=on
  LM_SpecialRoadType : Inport  Port=5  OutDataTypeStr=uint8  PortDimensions=1  BusOutputAsStruct=on
  LM_RoadNumChgType : Inport  Port=6  OutDataTypeStr=uint8  PortDimensions=1  BusOutputAsStruct=on
  LM_DrivInWLType : Inport  Port=7  OutDataTypeStr=uint8  PortDimensions=1  BusOutputAsStruct=on
  Bus Creator : BusCreator  Inputs=7
  Data Type Conversion : DataTypeConversion  OutDataTypeStr=Enum: LM_SpecialRoadType_E
  Data Type Conversion1 : DataTypeConversion  OutDataTypeStr=Enum: LM_RoadNumChg_E
  Data Type Conversion2 : DataTypeConversion  OutDataTypeStr=Enum: LM_DrivInWLFlag_E
  Data Type Conversion3 : DataTypeConversion  OutDataTypeStr=uint8
  Data Type Conversion4 : DataTypeConversion  OutDataTypeStr=uint8
  Data Type Conversion5 : DataTypeConversion  OutDataTypeStr=uint8
  LM_LL_Bus : Subsystem
  LM_LR_Bus : Subsystem
  LM_RL_Bus : Subsystem
  LM_RR_Bus : Subsystem
  Terminator : Terminator
  Terminator1 : Terminator
  Terminator2 : Terminator
  LM_SignalVerification : Outport
  wires:
  LM_LR_Bus/1(LM_LR_Bus) -> Bus Creator/2  "TOS_LM_LR_Bus"
  LM_RR_Bus/1(LM_RR_Bus) -> Bus Creator/4  "TOS_LM_RR_Bus"
  LM_RL_Bus/1(LM_RL_Bus) -> Bus Creator/3  "TOS_LM_RL_Bus"
  Data Type Conversion/1 -> Data Type Conversion5/1, Bus Creator/5  "TOS_PP_LM_SpecialRoadType"
  LM_LINE_LL/1 -> LM_LL_Bus/1(LM_LINE_LL)  "LM_LINE_LL"
  LM_LINE_RL/1 -> LM_RL_Bus/1(LM_LINE_RL)
  LM_LINE_RR/1 -> LM_RR_Bus/1(LM_LINE_RR)
  LM_LINE_LR/1 -> LM_LR_Bus/1(LM_LINE_LR)
  Data Type Conversion1/1 -> Data Type Conversion4/1, Bus Creator/6  "TOS_PP_LM_RoadNumChg"
  LM_LL_Bus/1(LM_LL_Bus) -> Bus Creator/1  "TOS_LM_LL_Bus"
  LM_SpecialRoadType/1 -> Data Type Conversion/1
  LM_DrivInWLType/1 -> Data Type Conversion2/1
  Data Type Conversion2/1 -> Data Type Conversion3/1, Bus Creator/7  "TOS_PP_LM_DrivInWLflg"
  LM_RoadNumChgType/1 -> Data Type Conversion1/1
  Data Type Conversion3/1 -> Terminator/1  "TOS_PP_LM_DrivInWLflg"
  Data Type Conversion4/1 -> Terminator1/1  "TOS_PP_LM_RoadNumChg"
  Data Type Conversion5/1 -> Terminator2/1  "TOS_PP_LM_SpecialRoadType"
  Bus Creator/1 -> LM_SignalVerification/1  "LM_SignalVerification"

== system PubIfDecisionTOS_MDL/TOS_20201112/TOS_2012080320/PP1128/ISV_InputSignalVerification/OFM_SignalVerif ==
  OFMInfo : Inport
  Bus Creator1 : BusCreator  Inputs=30
  Bus Selector : BusSelector  OutputSignals=Object_Fus_Type,Object_ID,Object_Type,Object_Length,Object_Width,Object_Hight,Object_HeadingAngle,Object_YawAngle,Object_MovingState,Object_Orientation,Object_DX,Object_DY,Object_VX,Object_VY,Object_Std_AX,Object_Std_AY,Object_Std_DX,Object_Std_DY,Object_Std_VX,Object_Std_VY,Object_AX,Object_AY,Object_Std_Length,Object_Std_Width,Object_Std_HeadingAngle,Object_Type_Prob,Object_ExistProb,Object_ObstacleProb,Object_Age
  Constant3 : Constant  Value=C_TOS_NumberOfEffectiveTargets  OutDataTypeStr=uint8
      settings: AttributesFormatString=C_TOS_NumberOfEffectiveTargets = 80
  Signal Copy{,1..27,30..31} (30 alike) : SignalConversion  OverrideOpt=off
  OFM_SignalVerification : Outport
  wires:
  Bus Selector/5 -> Signal Copy5/1  "<Object_Width>"
  Bus Selector/6 -> Signal Copy6/1  "<Object_Hight>"
  Signal Copy21/1 -> Bus Creator1/24  "Object_Std_Length"
  Bus Selector/13 -> Signal Copy13/1  "<Object_VX>"
  Bus Selector/12 -> Signal Copy12/1  "<Object_DY>"
  Signal Copy31/1 -> Bus Creator1/26  "Object_Std_HeadingAngle"
  Bus Selector/27 -> Signal Copy25/1  "<Object_ExistProb>"
  Bus Selector/9 -> Signal Copy9/1  "<Object_MovingState>"
  Signal Copy1/1 -> Bus Creator1/2  "Object_Fus_Type"
  Signal Copy15/1 -> Bus Creator1/16  "Object_Std_AX"
  Bus Selector/14 -> Signal Copy14/1  "<Object_VY>"
  Signal Copy12/1 -> Bus Creator1/13  "Object_DY"
  Signal Copy6/1 -> Bus Creator1/7  "Object_Hight"
  Bus Selector/10 -> Signal Copy10/1  "<Object_Orientation>"
  Signal Copy8/1 -> Bus Creator1/9  "Object_YawAngle"
  OFMInfo/1 -> Bus Selector/1
  Signal Copy30/1 -> Bus Creator1/25  "Object_Std_Width"
  Signal Copy5/1 -> Bus Creator1/6  "Object_Width"
  Bus Selector/17 -> Signal Copy23/1  "<Object_Std_DX>"
  Signal Copy27/1 -> Bus Creator1/30  "Object_Age"
  Bus Selector/18 -> Signal Copy16/1  "<Object_Std_DY>"
  Signal Copy25/1 -> Bus Creator1/28  "Object_ExistProb"
  Bus Selector/16 -> Signal Copy22/1  "<Object_Std_AY>"
  Signal Copy13/1 -> Bus Creator1/14  "Object_VX"
  Bus Selector/15 -> Signal Copy15/1  "<Object_Std_AX>"
  Bus Selector/21 -> Signal Copy19/1  "<Object_AX>"
  Bus Selector/22 -> Signal Copy20/1  "<Object_AY>"
  Signal Copy4/1 -> Bus Creator1/5  "Object_Length"
  Constant3/1 -> Signal Copy/1
  Bus Selector/3 -> Signal Copy3/1  "<Object_Type>"
  Signal Copy18/1 -> Bus Creator1/21  "Object_Std_VY"
  Bus Selector/1 -> Signal Copy1/1  "<Object_Fus_Type>"
  Signal Copy16/1 -> Bus Creator1/19  "Object_Std_DY"
  Bus Selector/29 -> Signal Copy27/1  "<Object_Age>"
  Signal Copy9/1 -> Bus Creator1/10  "Object_MovingState"
  Signal Copy24/1 -> Bus Creator1/27  "Object_Type_Prob"
  Bus Selector/23 -> Signal Copy21/1  "<Object_Std_Length>"
  Signal Copy14/1 -> Bus Creator1/15  "Object_VY"
  Bus Selector/26 -> Signal Copy24/1  "<Object_Type_Prob>"
  Bus Selector/25 -> Signal Copy31/1  "<Object_Std_HeadingAngle>"
  Signal Copy26/1 -> Bus Creator1/29  "Object_ObstacleProb"
  Bus Selector/2 -> Signal Copy2/1  "<Object_ID>"
  Signal Copy7/1 -> Bus Creator1/8  "Object_HeadingAngle"
  Signal Copy3/1 -> Bus Creator1/4  "Object_Type"
  Bus Selector/11 -> Signal Copy11/1  "<Object_DX>"
  Bus Selector/4 -> Signal Copy4/1  "<Object_Length>"
  Bus Selector/8 -> Signal Copy8/1  "<Object_YawAngle>"
  Signal Copy20/1 -> Bus Creator1/23  "Object_AY"
  Bus Selector/28 -> Signal Copy26/1  "<Object_ObstacleProb>"
  Signal Copy11/1 -> Bus Creator1/12  "Object_DX"
  Signal Copy2/1 -> Bus Creator1/3  "Object_ID"
  Bus Selector/20 -> Signal Copy18/1  "<Object_Std_VY>"
  Signal Copy10/1 -> Bus Creator1/11  "Object_Orientation"
  Bus Selector/19 -> Signal Copy17/1  "<Object_Std_VX>"
  Signal Copy/1 -> Bus Creator1/1  "Object_Num"
  Signal Copy22/1 -> Bus Creator1/17  "Object_Std_AY"
  Signal Copy19/1 -> Bus Creator1/22  "Object_AX"
  Signal Copy17/1 -> Bus Creator1/20  "Object_Std_VX"
  Bus Selector/7 -> Signal Copy7/1  "<Object_HeadingAngle>"
  Bus Creator1/1 -> OFM_SignalVerification/1
  Bus Selector/24 -> Signal Copy30/1  "<Object_Std_Width>"
  Signal Copy23/1 -> Bus Creator1/18  "Object_Std_DX"

== system PubIfDecisionTOS_MDL/TOS_20201112/TOS_2012080320/PP1128/ISV_InputSignalVerification/VIE_SignalVerif ==
  vxvRefMs : Inport
  psiDtOpt : Inport  Port=2  Interpolate=off
  kapTraj : Inport  Port=3
  axvRefMs2 : Inport  Port=4
  Bus Creator : BusCreator  Inputs=4
  Signal Copy{1..3,24} (4 alike) : SignalConversion  OverrideOpt=off
  VIE_SignalVerification : Outport
  wires:
  axvRefMs2/1 -> Signal Copy3/1
  vxvRefMs/1 -> Signal Copy24/1
  kapTraj/1 -> Signal Copy2/1
  psiDtOpt/1 -> Signal Copy1/1
  Bus Creator/1 -> VIE_SignalVerification/1
  Signal Copy24/1 -> Bus Creator/1  "vxvRefMs"
  Signal Copy1/1 -> Bus Creator/2  "psiDtOpt"
  Signal Copy2/1 -> Bus Creator/3  "kapTraj"
  Signal Copy3/1 -> Bus Creator/4  "axvRefMs2"

== system PubIfDecisionTOS_MDL/TOS_20201112/TOS_2012080320/TLJ/Pro/ObjInLane_Default ==
  Action Port : ActionPort  ActionPortLabel=if(u1 == 0)
  Constant1 : Constant  Value=0  OutDataTypeStr=boolean
  Constant2 : Constant  Value=0  OutDataTypeStr=boolean
  Constant3 : Constant  Value=0  OutDataTypeStr=boolean
  Constant4 : Constant  Value=0  OutDataTypeStr=single
  Constant5 : Constant  Value=0  OutDataTypeStr=single
  Constant6 : Constant  Value=0  OutDataTypeStr=single
  Constant7 : Constant  Value=0  OutDataTypeStr=uint8
  TLJ_ObjInLeftLane_flag : Outport
  TLJ_ObjInEgoLane_flag : Outport  Port=2
  TLJ_ObjInRightLane_flag : Outport  Port=3
  TOS_TLJ_ObjinLeftLaneProb_ObserVale : Outport  Port=4
  TOS_TLJ_ObjinEgoLaneProb_ObserVale : Outport  Port=5
  TOS_TLJ_ObjinRightLaneProb_ObserVale : Outport  Port=6
  TOS_TLJ_ObjInLaneCondition_Flag_ObserVale : Outport  Port=7
  wires:
  Constant3/1 -> TLJ_ObjInRightLane_flag/1  "ObjInRightLane_flag"
  Constant1/1 -> TLJ_ObjInLeftLane_flag/1  "ObjInLeftLane_flag"
  Constant2/1 -> TLJ_ObjInEgoLane_flag/1  "ObjInEgoLane_flag"
  Constant4/1 -> TOS_TLJ_ObjinLeftLaneProb_ObserVale/1
  Constant5/1 -> TOS_TLJ_ObjinEgoLaneProb_ObserVale/1
  Constant6/1 -> TOS_TLJ_ObjinRightLaneProb_ObserVale/1
  Constant7/1 -> TOS_TLJ_ObjInLaneCondition_Flag_ObserVale/1

== system PubIfDecisionTOS_MDL/TOS_20201112/TOS_2012080320/TLJ/Pro/Pro ==
  PIL_EgoLaneProb : Inport
  PIL_LeftLaneProb : Inport  Port=2
  PIL_RightLaneProb : Inport  Port=3
  PIL_EgoVehicle_EgoLaneProb : Inport  Port=4
  PIL_EgoVehicle_LeftLaneProb : Inport  Port=5
  PIL_EgoVehicle_RightLaneProb : Inport  Port=6
  Object_Type : Inport  Port=7
  Object_DY : Inport  Port=8
  PIL_CutinFlag : Inport  Port=9
  PIL_CutoutFlag : Inport  Port=10
  Action Port : ActionPort  ActionPortLabel=else
  Bus Creator : BusCreator  Inputs=10
  Bus Creator1 : BusCreator  Inputs=3
  Bus Selector : BusSelector  OutputSignals=PIL_EgoLaneProb,PIL_LeftLaneProb,PIL_RightLaneProb,PIL_EgoVehicle_EgoLaneProb,PIL_EgoVehicle_LeftLaneProb,PIL_EgoVehicle_RightLaneProb
  Bus Selector1 : BusSelector  OutputSignals=Object_Type,Object_DY,PIL_CutinFlag,PIL_CutoutFlag,PIL_EgoVehicle_LeftLaneProb,PIL_EgoVehicle_EgoLaneProb,PIL_EgoVehicle_RightLaneProb,PIL_LeftLaneProb,PIL_EgoLaneProb,PIL_RightLaneProb
  Bus Selector2 : BusSelector  OutputSignals=TLJ_ObjinLeftLaneProb,TLJ_ObjinEgoLaneProb,TLJ_ObjinRightLaneProb
  ObjInLane : Subsystem
  Pro : Subsystem
  TLJ_ObjInLeftLane_flag : Outport
  TLJ_ObjInEgoLane_flag : Outport  Port=2
  TLJ_ObjInRightLane_flag : Outport  Port=3
  TOS_TLJ_ObjinLeftLaneProb_ObserVale : Outport  Port=4
  TOS_TLJ_ObjinEgoLaneProb_ObserVale : Outport  Port=5
  TOS_TLJ_ObjinRightLaneProb_ObserVale : Outport  Port=6
  TOS_TLJ_ObjInLaneCondition_Flag_ObserVale : Outport  Port=7
  wires:
  PIL_EgoLaneProb/1 -> Bus Creator/1  "PIL_EgoLaneProb"
  PIL_LeftLaneProb/1 -> Bus Creator/2  "PIL_LeftLaneProb"
  PIL_RightLaneProb/1 -> Bus Creator/3  "PIL_RightLaneProb"
  PIL_EgoVehicle_EgoLaneProb/1 -> Bus Creator/4  "PIL_EgoVehicle_EgoLaneProb"
  PIL_EgoVehicle_LeftLaneProb/1 -> Bus Creator/5  "PIL_EgoVehicle_LeftLaneProb"
  PIL_EgoVehicle_RightLaneProb/1 -> Bus Creator/6  "PIL_EgoVehicle_RightLaneProb"
  PIL_CutinFlag/1 -> Bus Creator/9  "PIL_CutinFlag"
  Object_Type/1 -> Bus Creator/7  "Object_Type"
  Bus Creator/1 -> Bus Selector1/1, Bus Selector/1
  Bus Selector/1 -> Pro/1(PIL_EgoLaneProb)  "<PIL_EgoLaneProb>"
  Bus Selector/2 -> Pro/2(PIL_LeftLaneProb)  "<PIL_LeftLaneProb>"
  Bus Selector/3 -> Pro/3(PIL_RightLaneProb)  "<PIL_RightLaneProb>"
  Bus Selector/4 -> Pro/4(PIL_EgoVehicle_EgoLaneProb)  "<PIL_EgoVehicle_EgoLaneProb>"
  Bus Selector/5 -> Pro/5(PIL_EgoVehicle_LeftLaneProb)  "<PIL_EgoVehicle_LeftLaneProb>"
  Bus Selector/6 -> Pro/6(PIL_EgoVehicle_RightLaneProb)  "<PIL_EgoVehicle_RightLaneProb>"
  Bus Selector1/1 -> ObjInLane/1(Object_Type)  "<Object_Type>"
  Bus Selector1/3 -> ObjInLane/3(PIL_CutinFlag)  "<PIL_CutinFlag>"
  Bus Selector1/5 -> ObjInLane/5("PIL_EgoVehicleInLeftlaneProb  ")  "<PIL_EgoVehicle_LeftLaneProb>"
  Bus Selector1/6 -> ObjInLane/6("PIL_EgoVehicleInMiddlelaneProb  ")  "<PIL_EgoVehicle_EgoLaneProb>"
  Bus Selector1/7 -> ObjInLane/7("PIL_EgoVehicleInRightlaneProb  ")  "<PIL_EgoVehicle_RightLaneProb>"
  Bus Selector1/10 -> ObjInLane/10("PIL_ObjInRightlaneProb ")  "<PIL_RightLaneProb>"
  Pro/1(TLJ_ObjinLeftLaneProb) -> [TOS_TLJ_ObjinLeftLaneProb_ObserVale], Bus Creator1/1  "TLJ_ObjinLeftLaneProb"
  Pro/2(TLJ_ObjinEgoLaneProb) -> [TOS_TLJ_ObjinEgoLaneProb_ObserVale], Bus Creator1/2  "TLJ_ObjinEgoLaneProb"
  Pro/3(TLJ_ObjinRightLaneProb) -> [TOS_TLJ_ObjinRightLaneProb_ObserVale], Bus Creator1/3  "TLJ_ObjinRightLaneProb"
  Bus Creator1/1 -> Bus Selector2/1
  Bus Selector2/1 -> ObjInLane/11("TLJ_ObjinLeftLaneProb ")  "<TLJ_ObjinLeftLaneProb>"
  Bus Selector2/3 -> ObjInLane/13("TLJ_ObjInRightlaneProb ")  "<TLJ_ObjinRightLaneProb>"
  Bus Selector2/2 -> ObjInLane/12(TLJ_ObjinEgoLaneProb)  "<TLJ_ObjinEgoLaneProb>"
  ObjInLane/1(TLJ_ObjInLeftLane_flag) -> TLJ_ObjInLeftLane_flag/1
  ObjInLane/2(TLJ_ObjInEgoLane_flag) -> TLJ_ObjInEgoLane_flag/1
  ObjInLane/3(TLJ_ObjInRightLane_flag) -> TLJ_ObjInRightLane_flag/1
  Bus Selector1/8 -> ObjInLane/8("PIL_ObjinLeftLaneProb ")  "<PIL_LeftLaneProb>"
  Bus Selector1/9 -> ObjInLane/9(PIL_ObjinEgoLaneProb)  "<PIL_EgoLaneProb>"
  [TOS_TLJ_ObjinLeftLaneProb_ObserVale] -> TOS_TLJ_ObjinLeftLaneProb_ObserVale/1
  [TOS_TLJ_ObjinEgoLaneProb_ObserVale] -> TOS_TLJ_ObjinEgoLaneProb_ObserVale/1
  [TOS_TLJ_ObjinRightLaneProb_ObserVale] -> TOS_TLJ_ObjinRightLaneProb_ObserVale/1
  ObjInLane/4(TOS_TLJ_ObjInLaneCondition_Flag_ObserVale) -> [TOS_TLJ_ObjInLaneCondition_Flag_ObserVale]
  [TOS_TLJ_ObjInLaneCondition_Flag_ObserVale] -> TOS_TLJ_ObjInLaneCondition_Flag_ObserVale/1
  Object_DY/1 -> Bus Creator/8  "Object_DY"
  Bus Selector1/2 -> ObjInLane/2(Object_DY)  "<Object_DY>"
  PIL_CutoutFlag/1 -> Bus Creator/10  "PIL_CutoutFlag"
  Bus Selector1/4 -> ObjInLane/4(PIL_CutoutFlag)  "<PIL_CutoutFlag>"
